simulink model "PhipPoly"  (R2014b)
settings: Solver=ode45  StartTime=0.0  StopTime=10.0  RelTol=1e-3
values from neighbouring files (symbols this model uses):
  b = ku/k    [glabatom.m]
  C_norm = C / 16    [glabatom_pokus.m]
  delta = Jp*zeta*omegan    [glabatom.m]
  Jp = m*g*l/(omegan^2)    [glabatom.m]
undefined symbols (not defined in the file or in its folder): Alin, Blin, Clin, Dlin, k1, k2, k3, ku, up1, x1p, x2p, x3p, x4p, y1p, y2p
settings Model: Creator=glab  LastModifiedBy=glab

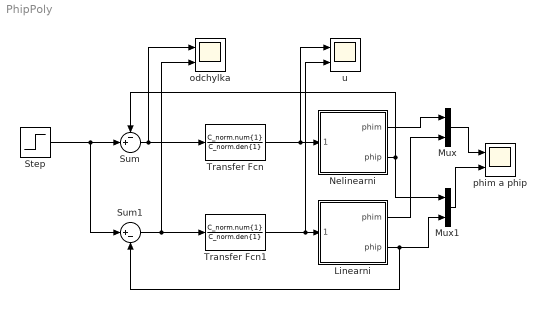
== system PhipPoly ==
  Linearni : Subsystem
  Mux : Mux  Inputs=2
  Mux1 : Mux  Inputs=2
  Nelinearni : Subsystem
  Step : Step  Time=0  After=-pi/2  SampleTime=0
  Sum : Sum  Inputs=-+|
  Sum1 : Sum  Inputs=|+-
  Transfer Fcn : TransferFcn  Numerator=C_norm.num{1}  Denominator=C_norm.den{1}
  Transfer Fcn1 : TransferFcn  Numerator=C_norm.num{1}  Denominator=C_norm.den{1}
  odchylka : Scope  NumInputPorts=2
      settings: ShowLegends=on  TimeRange=12.49629428456308  YMin=0.999999999999679~-1.570796326795069  YMax=0.9999999999998991~-1.570796326794724  SaveName=vystup2
  phim a phip : Scope  NumInputPorts=2
      settings: ShowLegends=on  TimeRange=12.49629428456308  YMin=0.999999999999679~-1.570796326795069  YMax=0.9999999999998991~-1.570796326794724  SaveName=vystup
  u : Scope  NumInputPorts=2
      settings: ShowLegends=on  TimeRange=12.49629428456308  YMin=0.999999999999679~-1.570796326795069  YMax=0.9999999999998991~-1.570796326794724  SaveName=vystup1
  wires:
  Mux1/1 -> phim a phip/2
  Linearni/2(phip) -> Mux1/2, Sum1/2
  Linearni/1(phim) -> Mux/2
  Nelinearni/2(phip) -> Mux1/1, Sum/1
  Step/1 -> Sum1/1, Sum/2
  Sum/1 -> Transfer Fcn/1, odchylka/1
  Sum1/1 -> Transfer Fcn1/1, odchylka/2
  Mux/1 -> phim a phip/1
  Nelinearni/1(phim) -> Mux/1
  Transfer Fcn/1 -> u/1, Nelinearni/1(u_norm)
  Transfer Fcn1/1 -> u/2, Linearni/1(u_norm)

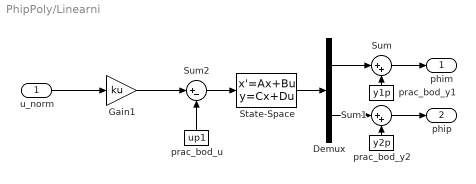
== system PhipPoly/Linearni ==
  u_norm : Inport
  Demux : Demux  Outputs=2
  Gain1 : Gain  Gain=ku
  State-Space : StateSpace  A=Alin  B=Blin  C=Clin  D=Dlin  X0=[0 pi/2 0 0]
  Sum : Sum  Inputs=|++
  Sum1 : Sum  Inputs=|++
  Sum2 : Sum  Inputs=|+-
  prac_bod_u : Constant  Value=up1
  prac_bod_y1 : Constant  Value=y1p
  prac_bod_y2 : Constant  Value=y2p
  phim : Outport
  phip : Outport  Port=2
  wires:
  State-Space/1 -> Demux/1
  Demux/1 -> Sum/1
  prac_bod_y1/1 -> Sum/2
  Sum/1 -> phim/1
  prac_bod_y2/1 -> Sum1/2
  Sum1/1 -> phip/1
  Demux/2 -> Sum1/1
  prac_bod_u/1 -> Sum2/2
  Sum2/1 -> State-Space/1
  u_norm/1 -> Gain1/1
  Gain1/1 -> Sum2/1

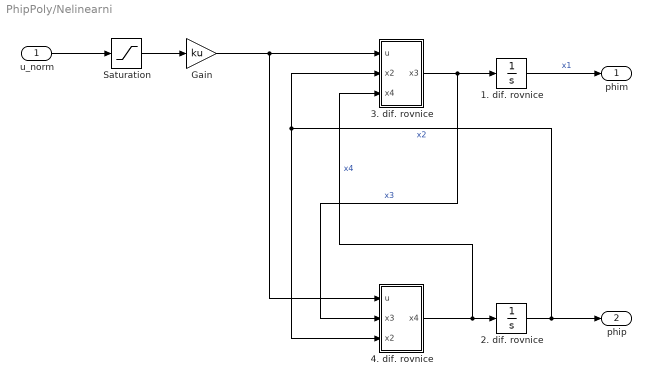
== system PhipPoly/Nelinearni ==
  u_norm : Inport
  1. dif. rovnice : Integrator  InitialCondition=x1p
  2. dif. rovnice : Integrator  InitialCondition=x2p
  3. dif. rovnice : Subsystem
  4. dif. rovnice : Subsystem
  Gain : Gain  Gain=ku
  Saturation : Saturate  UpperLimit=1  LowerLimit=-1
  phim : Outport
  phip : Outport  Port=2
  wires:
  1. dif. rovnice/1 -> phim/1  "x1"
  4. dif. rovnice/1(x4) -> 3. dif. rovnice/3(x4), 2. dif. rovnice/1  "x4"
  2. dif. rovnice/1 -> phip/1, 4. dif. rovnice/3(x2), 3. dif. rovnice/2(x2)  "x2"
  3. dif. rovnice/1(x3) -> 4. dif. rovnice/2("x3 "), 1. dif. rovnice/1  "x3"
  u_norm/1 -> Saturation/1
  Gain/1 -> 4. dif. rovnice/1(u), 3. dif. rovnice/1(u)
  Saturation/1 -> Gain/1

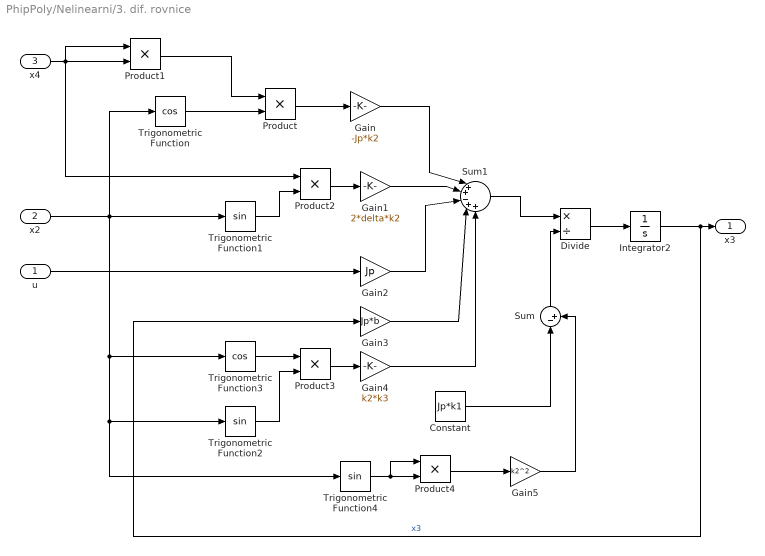
== system PhipPoly/Nelinearni/3. dif. rovnice ==
  u : Inport
  x2 : Inport  Port=2
  x4 : Inport  Port=3
  Constant : Constant  Value=Jp*k1
  Divide : Product  Inputs=*/
  Gain : Gain  Gain=-Jp*k2
  Gain1 : Gain  Gain=2*delta*k2
  Gain2 : Gain  Gain=Jp
  Gain3 : Gain  Gain=Jp*b
  Gain4 : Gain  Gain=k2*k3
  Gain5 : Gain  Gain=k2^2
  Integrator2 : Integrator  InitialCondition=x3p
  Product{,1..4} (5 alike) : Product
  Sum : Sum  Inputs=|-+
  Sum1 : Sum  Inputs=|++-++
  Trigonometric Function : Trigonometry  Operator=cos
  Trigonometric Function1 : Trigonometry
  Trigonometric Function2 : Trigonometry
  Trigonometric Function3 : Trigonometry  Operator=cos
  Trigonometric Function4 : Trigonometry
  x3 : Outport
  wires:
  Trigonometric Function3/1 -> Product3/1
  Divide/1 -> Integrator2/1
  x2/1 -> Trigonometric Function4/1, Trigonometric Function2/1, Trigonometric Function3/1, Trigonometric Function1/1, Trigonometric Function/1
  Product3/1 -> Gain4/1
  Trigonometric Function2/1 -> Product3/2
  Gain4/1 -> Sum1/5
  Gain/1 -> Sum1/1
  Product2/1 -> Gain1/1
  Trigonometric Function1/1 -> Product2/2
  u/1 -> Gain2/1
  Gain3/1 -> Sum1/4
  Gain1/1 -> Sum1/2
  Gain2/1 -> Sum1/3
  Sum1/1 -> Divide/1
  Product/1 -> Gain/1
  Sum/1 -> Divide/2
  x4/1 -> Product1/2, Product2/1, Product1/1
  Product1/1 -> Product/1
  Integrator2/1 -> Gain3/1, x3/1  "x3"
  Trigonometric Function/1 -> Product/2
  Gain5/1 -> Sum/2
  Constant/1 -> Sum/1
  Product4/1 -> Gain5/1
  Trigonometric Function4/1 -> Product4/1, Product4/2

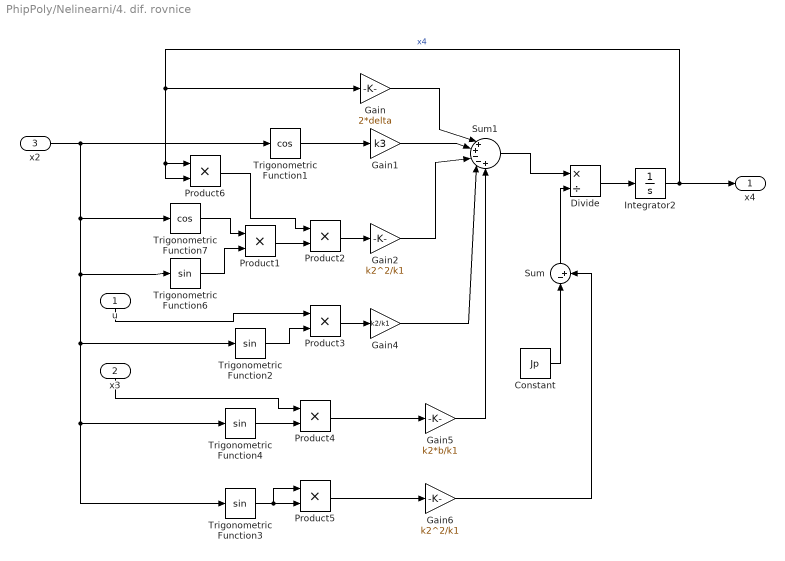
== system PhipPoly/Nelinearni/4. dif. rovnice ==
  u : Inport
  "x3 " : Inport  Port=2
  x2 : Inport  Port=3
  Constant : Constant  Value=Jp
  Divide : Product  Inputs=*/
  Gain : Gain  Gain=2*delta
  Gain1 : Gain  Gain=k3
  Gain2 : Gain  Gain=k2^2/k1
  Gain4 : Gain  Gain=k2/k1
  Gain5 : Gain  Gain=k2*b/k1
  Gain6 : Gain  Gain=k2^2/k1
  Integrator2 : Integrator  InitialCondition=x4p
  Product{1..6} (6 alike) : Product
  Sum : Sum  Inputs=|-+
  Sum1 : Sum  Inputs=|++--+
  Trigonometric Function1 : Trigonometry  Operator=cos
  Trigonometric Function{2..4,6} (4 alike) : Trigonometry
  Trigonometric Function7 : Trigonometry  Operator=cos
  x4 : Outport
  wires:
  Trigonometric Function3/1 -> Product5/1, Product5/2
  Product5/1 -> Gain6/1
  Divide/1 -> Integrator2/1
  Product3/1 -> Gain4/1
  Gain/1 -> Sum1/1
  Constant/1 -> Sum/1
  Gain6/1 -> Sum/2
  Integrator2/1 -> x4/1, Gain/1, Product6/1, Product6/2  "x4"
  Sum/1 -> Divide/2
  Product4/1 -> Gain5/1
  Sum1/1 -> Divide/1
  Gain2/1 -> Sum1/3
  Gain1/1 -> Sum1/2
  Trigonometric Function1/1 -> Gain1/1
  Trigonometric Function2/1 -> Product3/2
  Trigonometric Function6/1 -> Product1/2
  Trigonometric Function7/1 -> Product1/1
  Gain5/1 -> Sum1/5
  Trigonometric Function4/1 -> Product4/2
  Gain4/1 -> Sum1/4
  Product2/1 -> Gain2/1
  u/1 -> Product3/1
  x2/1 -> Trigonometric Function3/1, Trigonometric Function4/1, Trigonometric Function2/1, Trigonometric Function6/1, Trigonometric Function7/1, Trigonometric Function1/1
  "x3 "/1 -> Product4/1
  Product1/1 -> Product2/2
  Product6/1 -> Product2/1
